simulink model "servomotor_posicao_Kalman_Com_Ruido_Posicao"  (R2024b)
settings: Solver=FixedStepAuto  StartTime=0.0  StopTime=tf  FixedStep=1e-6  RelTol=1e-3
values from neighbouring files (symbols this model uses):
  controlador =     [controlador.mat]    (also in projetarControladorPosicaoOtimizacao.m = projetarControladorPosicaoAnalitico(requisitos, planta))
  planta =     [controlador.mat]    (also in kalman.m = obterPlantaServoPosicao())
  var_theta = 1    [avaliarQuantizacao_Kalman_Com_Ruido_Posicao.m]    (also in avaliarQuantizacao_PB_Com_Ruido_Posicao.m; simularRespostaDegrau_EKF_Com_Ruido.m = var_thetas(i); simularRespostaDegrau_Kalman_Com_Ruido.m = var_thetas(i); simularRespostaDegrau_PB_Com_Ruido.m = var_thetas(i))
undefined symbols (not defined in the file or in its folder): Discrete, Time
libraries: ctrlSharedLib x1
settings Model: Creator=mmaximo  LastModifiedBy=dibue
settings SolverCC: AlgebraicLoopSolver=TrustRegion
settings DebuggingCC: UnconnectedInputMsg=warning  UnconnectedOutputMsg=warning  UnconnectedLineMsg=warning
settings ModelReferenceCC: EnableRefExpFcnMdlSchedulingChecks=on
settings RTWCC: GPUComputeCapability=3.5

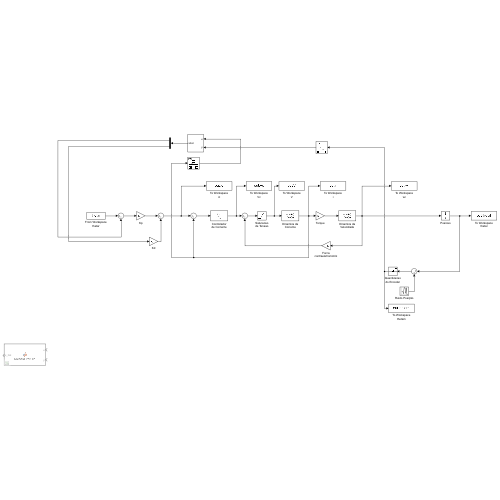
[thumbnail: Simulink's stored preview of the top-level diagram]
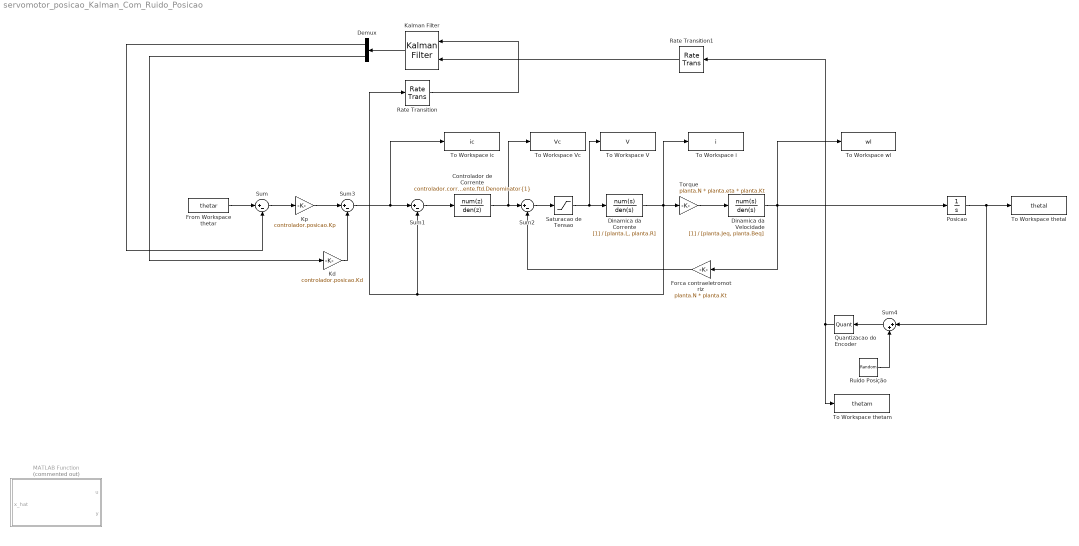
== system servomotor_posicao_Kalman_Com_Ruido_Posicao ==
  Controlador de Corrente : DiscreteTransferFcn  Numerator=controlador.corrente.ftd.Numerator{1}  Denominator=controlador.corrente.ftd.Denominator{1}  SampleTime=controlador.corrente.T
  Demux : Demux  Outputs=2
  Dinamica da Corrente : TransferFcn  Denominator=[planta.L, planta.R]
  Dinamica da Velocidade : TransferFcn  Denominator=[planta.Jeq, planta.Beq]
  Forca contraeletromotriz : Gain  Gain=planta.N * planta.Kt
  From Workspace thetar : FromWorkspace  VariableName=thetar
  Kalman Filter : ctrlSharedLib/Kalman Filter  TimeDomain=Discrete-Time  UseCurrentEstimator=on  ModelSource=Individual A, B, C, D matrices  ModelSourceVariable=ss(0.95,1,1,0,1)  A=planta.Kalman.A  B=planta.Kalman.B  C=planta.Kalman.C  D=planta.Kalman.D  NumberOfStates=1  NumberOfInputs=1  NumberOfOutputs=1  InitialEstimateSource=Dialog  X0=0  P0=10  UseK=off  UseGH=off  NumberOfProcessNoiseInputs=1  G=1  TimeInvariantG=on  H=0  TimeInvariantH=on  Q=planta.Kalman.Q  TimeInvariantQ=on  R=planta.Kalman.R  TimeInvariantR=on  N=0  TimeInvariantN=on  AddInputPort=on  AddEnablePort=off  OutputEstimatedY=off  OutputP=off  Ts=-1
  Kd : Gain  Gain=controlador.posicao.Kd
  Kp : Gain  Gain=controlador.posicao.Kp
  MATLAB Function : MATLAB Function  Commented=on  TreatAsAtomicUnit=on
  Posicao : Integrator
  Quantizacao do Encoder : Quantizer  QuantizationInterval=planta.quantizacaoEncoder
  Rate Transition : RateTransition  OutPortSampleTime=controlador.posicao.T
  Rate Transition1 : RateTransition  OutPortSampleTime=controlador.posicao.T
  Ruido Posição : RandomNumber  Tag=Ruido_posicao  Description=Ruido_posicao  Variance=var_theta  SampleTime=0.01
  Saturacao de Tensao : Saturate  UpperLimit=planta.Vmax  LowerLimit=-planta.Vmax
  Sum{,1..3} (4 alike) : Sum  Inputs=|+-
  Sum4 : Sum  Inputs=|++
  To Workspace V : ToWorkspace  VariableName=V  SaveFormat=Structure With Time  SampleTime=1e-6
  To Workspace Vc : ToWorkspace  VariableName=Vc  SaveFormat=Structure With Time  SampleTime=1e-6
  To Workspace i : ToWorkspace  VariableName=i  SaveFormat=Structure With Time  SampleTime=1e-6
  To Workspace ic : ToWorkspace  VariableName=ic  SaveFormat=Structure With Time  SampleTime=1e-6
  To Workspace thetal : ToWorkspace  VariableName=thetal  SaveFormat=Structure With Time  SampleTime=-1
  To Workspace thetam : ToWorkspace  VariableName=thetam  SaveFormat=Structure With Time  SampleTime=-1
  To Workspace wl : ToWorkspace  VariableName=wl  SaveFormat=Structure With Time  SampleTime=1e-6
  Torque : Gain  Gain=planta.N * planta.eta * planta.Kt
  wires:
  From Workspace thetar/1 -> Sum/1
  Dinamica da Velocidade/1 -> To Workspace wl/1, Forca contraeletromotriz/1, Posicao/1
  Torque/1 -> Dinamica da Velocidade/1
  Forca contraeletromotriz/1 -> Sum2/2
  Sum1/1 -> Controlador de Corrente/1
  Sum/1 -> Kp/1
  Posicao/1 -> Sum4/1, To Workspace thetal/1
  Quantizacao do Encoder/1 -> To Workspace thetam/1, Rate Transition1/1
  Dinamica da Corrente/1 -> To Workspace i/1, Torque/1, Rate Transition/1, Sum1/2
  Kp/1 -> Sum3/1
  Sum3/1 -> To Workspace ic/1, Sum1/1
  Demux/1 -> Sum/2
  Ruido Posição/1 -> Sum4/2
  Saturacao de Tensao/1 -> To Workspace V/1, Dinamica da Corrente/1
  Sum2/1 -> Saturacao de Tensao/1
  Controlador de Corrente/1 -> To Workspace Vc/1, Sum2/1
  Demux/2 -> Kd/1
  Kd/1 -> Sum3/2
  Sum4/1 -> Quantizacao do Encoder/1
  Kalman Filter/1 -> Demux/1
  Rate Transition/1 -> Kalman Filter/1
  Rate Transition1/1 -> Kalman Filter/2

== matlab function servomotor_posicao_Kalman_Com_Ruido_Posicao/MATLAB Function ==
  data: u input; x_hat output; y input; planta parameter
function x_hat = KalmanFilterFcn(u, y, planta)
% KalmanFilterFcn: Implements a discrete Kalman Filter from a continuous plant model.
%   u: Control input vector
%   y: Measurement output vector

persistent x_hat_prev u_prev P_prev A B C D Q R;

A = planta.Kalman.A;
B = planta.Kalman.B;
C = planta.Kalman.C;
D = planta.Kalman.D;
Q = planta.Kalman.Q;
R = planta.Kalman.R;


% Initialization
if isempty(x_hat_prev)
    x_hat_prev = zeros(size(A, 1), 1);
    P_prev = eye(size(A, 1));
    u_prev = 0;
end

% --- Kalman Filter Prediction Step ---
% Propagate state estimate (x_hat_minus is the predicted state before measurement)
x_hat_minus = A * x_hat_prev + B * u;

% Propagate error covariance (P_minus is the predicted covariance before measurement)
P_minus = A * P_prev * A' + Q;

% --- Kalman Filter Update Step ---
% Calculate Kalman Gain
S = C * P_minus * C' + R; % Innovation (or residual) covariance
K = S \ (P_minus * C'); % Kalman Gain

% Update state estimate (incorporate measurement)
y_pred = C * x_hat_minus + D * u_prev; % Predicted measurement
innovation = y - y_pred;       % Measurement residual
x_hat_plus = x_hat_minus + K * innovation;

% Update error covariance
I = eye(size(P_minus));
P_plus = (I - K * C) * P_minus *(I - K * C)' + K*R*K';

% --- Store updated state and covariance for the next iteration ---
x_hat_prev = x_hat_plus;
u_prev = u;
P_prev = P_plus;

% --- Output the current state estimate ---
x_hat = x_hat_plus;

end
